simulink model "SailingYachtModel"  (R2022b)
settings: Solver=ode3  StartTime=0.0  StopTime=250  FixedStep=0.05  RelTol=1e-3  EnableMultiTasking=on
undefined symbols (not defined in the file or in its folder): par, Waypoints
libraries: simulink x1, vrlib x1
settings Model: Creator=Administrator  LastModifiedBy=ruben
settings SolverCC: AlgebraicLoopSolver=TrustRegion  AutoInsertRateTranBlk=on
settings DataIOCC: LimitDataPoints=on  SaveFormat=Array  SignalLoggingSaveFormat=ModelDataLogs  ReturnWorkspaceOutputs=off
settings OptimizationCC: ExpressionDepthLimit=2147483647  InitFltsAndDblsToZero=on  LifeSpan=inf
settings DebuggingCC: SaveWithParameterizedLinksMsg=none  UnderspecifiedInitializationDetection=Classic  MergeDetectMultiDrivingBlocksExec=none  SignalResolutionControl=TryResolveAllWithWarning  SolverPrmCheckMsg=warning  MultiTaskDSMMsg=warning  MultiTaskCondExecSysMsg=none  FcnCallInpInsideContextMsg=warning  UnconnectedInputMsg=warning  UnconnectedOutputMsg=warning  UnconnectedLineMsg=warning  StateNameClashWarn=warning  SFUnexpectedBacktrackingDiag=warning  SFNoUnconditionalDefaultTransitionDiag=warning  SFExecutionAtInitializationDiag=none  SFMachineParentedDataDiag=warning  ArithmeticOperatorsInVariantConditions=warning
settings HardwareCC: ProdBitPerPointer=32  ProdBitPerSizeT=32  ProdBitPerPtrDiffT=32  ProdLargestAtomicFloat=None  ProdIntDivRoundTo=Undefined  ProdEndianess=Unspecified  ProdWordSize=32  ProdHWDeviceType=32-bit Generic
settings ModelReferenceCC: PropagateSignalLabelsOutOfModel=off
settings SFSimCC: SimUseLocalCustomCode=off  CustomCodeUndefinedFunction=UseInterfaceOnly
settings RTWCC: RTWUseLocalCustomCode=off
settings CodeAppCC: StateflowObjectComments=on
settings GRTTargetCC: TargetFcnLib=ansi_tfl_tmw.mat  TargetLangStandard=C89/C90 (ANSI)  CombineOutputUpdateFcns=off  GRTInterface=on
settings ConfigComp: CovMetricSettings=dw  CovSaveCumulativeToWorkspaceVar=on  CovSaveSingleToWorkspaceVar=on  CovExternalEMLEnable=off

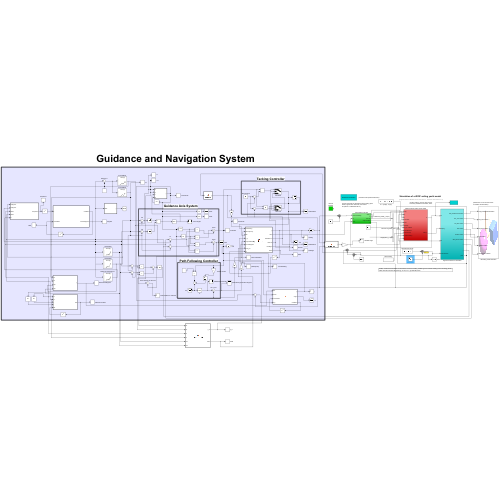
[thumbnail: Simulink's stored preview of the top-level diagram]
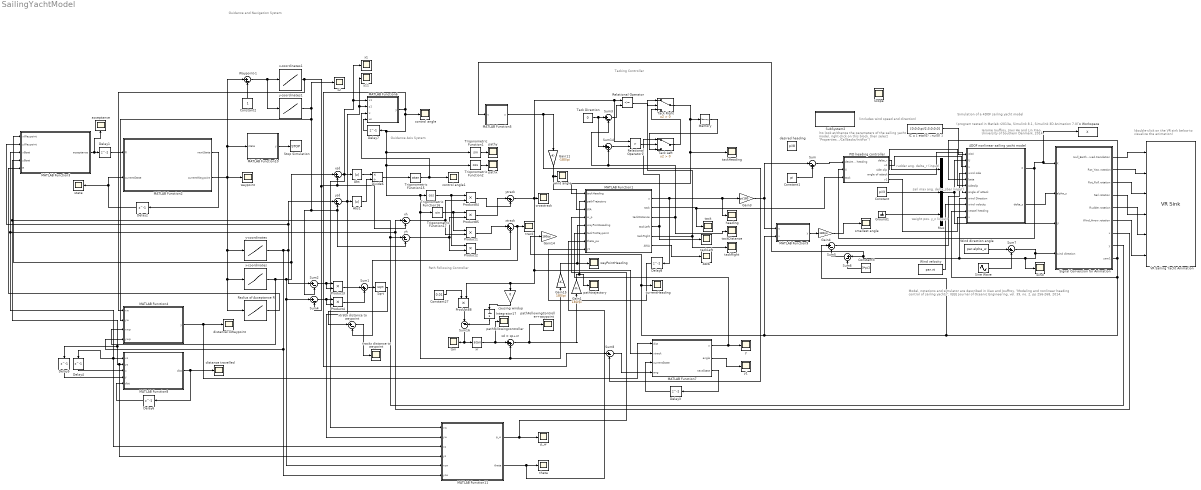
== system SailingYachtModel ==
  note: Guidance Axis System
  note: (includes wind speed and direction)
  note: (program tested in Matlab r2013a, Simulink 8.1, Simulink 3D Animation 7.0)
  note: (double-click on the VR sink below
      | to visualize the animation)
  note: Jerome Jouffroy, Jiaxi He and Lin Xiao,
      | University of Southern Denmark, 2014.
  note: Model, notations and simulator are described in Xiao and Jouffroy, "Modeling and nonlinear heading control of sailing yachts",
      | IEEE Journal of Oceanic Engineering, vol. 39, no. 2, pp 256-268, 2014.
  note: (to look at/change the parameters of the sailing yacht
      | model, right-click on this block, then select
      | "Properties.../Callbacks/InitFcn")
  note: weight pos. y_c (input)
  note: rudder ang. delta_r (input)
  note: sail max ang. delta_sbar (input)
  note: Simulation of a 4DOF sailing yacht model
  note: Path Following Controller
  note: Tacking Controller
  note: Guidance and Navigation System
  4DOF nonlinear sailing yacht model : Subsystem
  AWA : Scope
  Abs : Abs  SaturateOnIntegerOverflow=off
  Abs1 : Abs  SaturateOnIntegerOverflow=off
  Constant : Constant  Value=pi/3
  Constant1 : Constant  Value=pi
  Constant2 : Constant
  Constant27 : Constant  Value=0.01
  Constant3 : Constant  Value=3*pi/2
  Delay{1..8} (8 alike) : Delay  DelayLength=1
  Divide6 : Product  Inputs=*/
  Gain{1,4,14..15} (4 alike) : Gain  Gain=180/pi
  Gain11 : Gain  Gain=-180/pi
  Gain3 : Gain  Gain=pi/180
  Ground1 : Ground
  IC = [ eta(0) ; nu(0) ] : Constant  Value=[0;0;0;pi/2;3;0;0;0]
  Integrator17 : Integrator  LimitOutput=on  UpperSaturationLimit=10  LowerSaturationLimit=-10
  MATLAB Function1 : MATLAB Function  TreatAsAtomicUnit=on
  MATLAB Function10 : MATLAB Function  TreatAsAtomicUnit=on
  MATLAB Function11 : MATLAB Function  TreatAsAtomicUnit=on
  MATLAB Function2 : MATLAB Function  TreatAsAtomicUnit=on
  MATLAB Function3 : MATLAB Function  TreatAsAtomicUnit=on
  MATLAB Function4 : MATLAB Function  TreatAsAtomicUnit=on
  MATLAB Function5 : MATLAB Function  TreatAsAtomicUnit=on
  MATLAB Function6 : MATLAB Function  TreatAsAtomicUnit=on
  MATLAB Function7 : MATLAB Function  TreatAsAtomicUnit=on
  MATLAB Function8 : MATLAB Function  TreatAsAtomicUnit=on
  MATLAB Function9 : MATLAB Function  TreatAsAtomicUnit=on
  Memory : Memory
  Mux : Mux  Inputs=3
  PID heading controller : Subsystem
  Product{1..4,84..85,88} (7 alike) : Product
  Radius of Acceptance R : Lookup_n-D  NumberOfTableDimensions=1  BreakpointsForDimension1=Waypoints.number  Table=Waypoints.R  InterpMethod=Cubic spline  ExtrapMethod=Cubic spline  InternalRulePriority=Speed  RndMeth=Simplest
  Relational Operator : RelationalOperator  Operator=<=  OutDataTypeStr=boolean  RndMeth=Simplest  InputSameDT=off
  Relational Operator1 : RelationalOperator  Operator=>  OutDataTypeStr=boolean  RndMeth=Simplest  InputSameDT=off
  Signal Conversion for Animation : Subsystem
  Sine Wave : Sin  Amplitude=pi/14  Frequency=0.1  SampleTime=0
  Sqrt : Sqrt
  Stop Simulation : Stop
  SubSystem2 : Subsystem  InitFcn=|
      | global par
      | par.m = 25900;                         % (kg),mass of the vehicle
      | par.Ixx = 133690;          
      | par.Izz = 24760;      
      | par.Ixz = 2180;                        % moment of inertia
      | par.a11 = 970;   
      | par.a22 = 17430; 
      | par.a44 = 106500;
      | par.a66 = 101650;
      | par.a24 = -13160;
      | par.a26 = -6190; 
      | par.a46 = 4730;                        % (kg),added mass coef.
      | 
      | par.vt = 15;                           % the norm of wind velocity
      | par.alpha_w = -(-pi/2+pi/18);                      % the direction of wind (coming from the north, ie going south)
      | 
      | par.rho_a = 1.2;                       % (kg/m^3), air density
      | par.As = 170;                          % (m^2), sail area
      | par.h0 = 0.0005;                       % (m), roughness height
      | par.h1 = 11.58;                        % (m), reference height
      | par.z_s = -11.58;                      % (m), (x,y,z) is the CoE
      | par.xs = 0;
      | par.ys = 0;
      | par.zs = -11.58;                       % (m), (x,y,z) is the CoE
      | par.Xce = 0.6;                         % (m), distance along the mast to the CoE
      | par.Xm = 0.3;                          % (m), x-coordinate of the mast 
      | 
      | par.rho_w = 1025;                      % (kg/m^3), water density
      | par.Ar = 1.17;                         % (m^2), rudder area
      | par.d_r = 1.9;                         % rudder draft
      | par.zeta_r = 0.8;                      % rudder efficiency
      | par.x_r = -8.2;
      | par.z_r = -0.78;                       % (m), (x,y,z) is the CoE
      | par.xr = -8.2;
      | par.yr = 0;
      | par.zr = -0.78;                        % (m), (x,y,z) is the CoE
      | 
      | par.Ak = 8.7;                          % (m^2), keel area
      | par.d_k = 2.49;                        % keel draft
      | par.zeta_k = 0.7;                      % keel efficiency
      | par.x_k = 0;
      | par.z_k = -0.58;                       % (m), (x,y,z) is the CoE
      | par.xk = 0;
      | par.yk = 0;
      | par.zk = -0.58;                        % (m), (x,y,z) is the CoE
      | 
      | par.x_h = 0;
      | par.z_h = -1.18;                       % (m), (x,y,z) is the CoE
      | par.xh = 0;
      | par.yh = 0;
      | par.zh = -1.18;                        % (m), (x,y,z) is the CoE
      | 
      | par.w_c = 60000;                       % (N), crew weight 20000
      | par.x_c = -8;                          % (m), crew position
      | par.y_bm = 3.6;                        % (m), yacht beam
      | 
      | par.a = -5.89;
      | par.b = 8160;
      | par.c = 120000;
      | par.d = 50000;
      mask Display: disp('Parameter Initialization')
  Sum : Sum  Inputs=|-+  SaturateOnIntegerOverflow=on
  Sum1 : Sum  Inputs=|++
  Sum14 : Sum  Inputs=|++
  Sum16 : Sum  Inputs=|--
  Sum{2..4,8} (4 alike) : Sum  Inputs=|+-
  Sum5 : Sum  Inputs=|+-  SaturateOnIntegerOverflow=on
  Sum6 : Sum  Inputs=|+-  SaturateOnIntegerOverflow=on
  Sum7 : Sum  Inputs=|+-  SaturateOnIntegerOverflow=on
  Tack Direction : Constant  Value=0
  Tack Left : Switch  Criteria=u2 > Threshold  SaturateOnIntegerOverflow=off  InputSameDT=off
  Tack Right : Switch  Criteria=u2 > Threshold  SaturateOnIntegerOverflow=off  InputSameDT=off
  To Workspace : ToWorkspace  VariableName=X  SaveFormat=Structure With Time  SampleTime=-1
  Trigonometric Function1 : Trigonometry
  Trigonometric Function15 : Trigonometry  Operator=atan
  Trigonometric Function16 : Trigonometry  Operator=cos
  Trigonometric Function17 : Trigonometry
  Trigonometric Function2 : Trigonometry  Operator=cos
  VR Sailing Yacht Animation : vrlib/VR Sink  InstantiateOnLoad=on  SampleTime=-1  ViewEnable=on  RemoteChange=off  RemoteView=off  FieldsWritten=Hull_EarthFixed.translation.3.1.1.double#Rot_Yaw.rotation.4.1.1.double#Rot_Roll.rotation.4.1.1.double#Sail.rotation.4.1.1.double#Rudder.rotation.4.1.1.double#Wind_Arrow.rotation.4.1.1.double  WorldFileName=SailingYachtAnimation.wrl  WorldDescription=Sailing Yacht VR animation  AutoView=on  VideoDimensions=[]  AllowVariableSize=off  FigureProperties="{'Position', 'Name', 'Viewpoint', 'CameraBound', 'CameraDirection', 'CameraPosition', 'CameraUpVector', 'ZoomFactor', 'Antialiasing', 'Headlight', 'Lighting', 'NavPanel', 'Sound', 'StatusBar', 'Stereo3D', 'Stereo3DCameraOffset', 'Stereo3DHIT', 'ToolBar', 'Textures', 'Transparency', 'Triad', 'Wireframe', 'NavZones', 'NavMode', 'NavSpeed', 'CaptureFileFormat', 'CaptureFileName', 'Record2DCompressMethod', 'Record2DCompressQuality', 'Record2D', 'Record2DFileName', 'Record2DFPS'; [2.0000000000000000e+00   8.4000000000000000e+01   9.5800000000000000e+02   8.9600000000000000e+02], 'Sailing Yacht VR animation', 'Stern', 'on', [2.8705425156036607e-01   0.0000000000000000e+00  -9.5791432636803509e-01], [-1.9182625747857539e+01   1.3000000000000000e+01   3.6417716435568920e+01], [0.0000000000000000e+00   1.0000000000000000e+00   0.0000000000000000e+00], [1.0000000000000000e+00], 'on', 'on', 'on', 'halfbar', 'on', 'on', 'off', [1.0000000149011612e-01], [0.0000000000000000e+00], 'on', 'on', 'on', 'none', 'off', 'off', 'walk', 'normal', 'tif', '%f_anim_%n.tif', 'auto', [7.5000000000000000e+01], 'on', '%f_anim_%n.avi', [1.5000000000000000e+01]}"
  Waypoint-1 : Sum  Inputs=|+-
  Wind direction angle : Constant  Value=par.alpha_w
  Wind velocity : Constant  Value=par.vt
  acceptance : Scope
  causing windup : Gain  Gain=0
  control angle : Scope
  control angle1 : Scope
  crosstrack : Scope
  currentHeading : Scope
  desired heading : Constant  Value=pi/8
  distance travelled : Scope
  distanceToWaypoint : Scope
  heading : Scope
  p_w : Scope
  "pathFollowingController+waypoint " : Scope
  pathfollowingcontroller : Scope
  pathtrajectory : Scope
  pathx : Scope
  pathy : Scope
  smallest angle : Scope
  state : Scope
  tack : Scope
  tackDistance : Scope
  tackHeading : Scope
  tackLeft : Scope
  tackRight : Scope
  tan : Scope
  theta : Scope
  track : Scope
  trackx distance to waypoint : Scope
  wayPointHeading : Scope
  waypoint : Scope
  wind : Scope
  wind angle : Scope
  x-coordinates : Lookup_n-D  NumberOfTableDimensions=1  BreakpointsForDimension1=Waypoints.number  Table=Waypoints.x  InterpMethod=Cubic spline  ExtrapMethod=Cubic spline  InternalRulePriority=Speed  RndMeth=Simplest
  x-coordinates1 : Lookup_n-D  NumberOfTableDimensions=1  BreakpointsForDimension1=Waypoints.number  Table=Waypoints.x  InterpMethod=Cubic spline  ExtrapMethod=Cubic spline  InternalRulePriority=Speed  RndMeth=Simplest
  x1 : Scope
  x2 : Scope
  xd = xp+xr : Sum  Inputs=|++
  xh : Sum  Inputs=|+-
  xr : Trigonometry  Operator=atan
  xsd : Sum  Inputs=|+-
  xtrack : Sum  Inputs=|++
  xtrack distance to waypoint : Sum  Inputs=|+-
  y : Scope
  y-coordinates : Lookup_n-D  NumberOfTableDimensions=1  BreakpointsForDimension1=Waypoints.number  Table=Waypoints.y  InterpMethod=Cubic spline  ExtrapMethod=Cubic spline  InternalRulePriority=Speed  RndMeth=Simplest
  y-coordinates1 : Lookup_n-D  NumberOfTableDimensions=1  BreakpointsForDimension1=Waypoints.number  Table=Waypoints.y  InterpMethod=Cubic spline  ExtrapMethod=Cubic spline  InternalRulePriority=Speed  RndMeth=Simplest
  y1 : Scope
  y11 : Scope
  yh : Sum  Inputs=|+-
  ysd : Sum  Inputs=|+-
  ytrack : Sum  Inputs=|-+
  Scope : Scope
  wires:
  Constant/1 -> Mux/2
  IC = [ eta(0) ; nu(0) ]/1 -> 4DOF nonlinear sailing yacht model/1(X(0))
  Mux/1 -> Signal Conversion for Animation/3(U), 4DOF nonlinear sailing yacht model/2(U)
  4DOF nonlinear sailing yacht model/1(X) -> Signal Conversion for Animation/1(X), To Workspace/1, PID heading controller/2(X)
  PID heading controller/1(delta_r) -> Mux/1
  Ground1/1 -> Mux/3
  4DOF nonlinear sailing yacht model/2(delta_s) -> Signal Conversion for Animation/2(alpha_s)
  Signal Conversion for Animation/1(Hull_EarthFixed.translation) -> VR Sailing Yacht Animation/1
  Signal Conversion for Animation/2(Rot_Yaw.rotation) -> VR Sailing Yacht Animation/2
  Signal Conversion for Animation/4(Sail.rotation) -> VR Sailing Yacht Animation/4
  Signal Conversion for Animation/3(Rot_Roll.rotation) -> VR Sailing Yacht Animation/3
  Signal Conversion for Animation/5(Rudder.rotation) -> VR Sailing Yacht Animation/5
  Signal Conversion for Animation/6(Wind_Arrow.rotation) -> VR Sailing Yacht Animation/6
  Delay1/1 -> MATLAB Function2/1(R)
  Delay2/1 -> MATLAB Function2/2(currentState), state/1
  Trigonometric Function15/1 -> control angle1/1, MATLAB Function6/3(u)
  ysd/1 -> MATLAB Function11/2(yw), y11/1, MATLAB Function6/2(y1), Abs1/1
  Trigonometric Function17/1 -> Product1/1, Product85/1
  Product85/1 -> ytrack/1
  Product84/1 -> ytrack/2
  Trigonometric Function16/1 -> Product2/1, Product84/1
  xh/1 -> Product84/2, Product1/2
  xsd/1 -> MATLAB Function11/1(xw), MATLAB Function6/1(x1), x1/1, Abs/1
  yh/1 -> Product85/2, Product2/2
  Divide6/1 -> Trigonometric Function15/1
  MATLAB Function2/2(currentWaypoint) -> MATLAB Function10/1(state), Waypoint-1/1, waypoint/1, Radius of Acceptance R/1, x-coordinates/1, y-coordinates/1
  Waypoint-1/1 -> x-coordinates1/1, y-coordinates1/1
  Constant2/1 -> Waypoint-1/2
  MATLAB Function2/1(nextState) -> Delay2/1
  y-coordinates/1 -> MATLAB Function11/6(ycw), MATLAB Function4/4(ywp), MATLAB Function3/2(yWaypoint), ysd/1, Sum2/1
  x-coordinates/1 -> MATLAB Function4/3(xwp), MATLAB Function11/5(xcw), Sum4/1, xsd/1, MATLAB Function3/1(xWaypoint)
  y-coordinates1/1 -> MATLAB Function4/2(yw), yh/2, ysd/2, Sum2/2, x2/1
  x-coordinates1/1 -> MATLAB Function4/1(xw), Sum4/2, xh/2, xsd/2
  MATLAB Function6/1(y) -> Trigonometric Function1/1, Trigonometric Function2/1, Trigonometric Function17/1, xd = xp+xr/2, Gain15/1, Trigonometric Function16/1, Delay7/1, control angle/1, Sum8/1
  Product88/1 -> Sum16/1
  Sum16/1 -> xr/1, tan/1
  Constant27/1 -> Product88/1
  xr/1 -> xd = xp+xr/1, pathfollowingcontroller/1
  Gain15/1 -> MATLAB Function1/5(wayPointHeading), wayPointHeading/1
  Signal Conversion for Animation/7(x) -> xh/1, MATLAB Function11/3(xs), MATLAB Function8/1(xs), Delay4/1, MATLAB Function3/3(xBoat)
  Signal Conversion for Animation/8(y) -> yh/1, MATLAB Function3/4(yBoat), MATLAB Function11/4(ys), MATLAB Function8/2(ys), Delay5/1
  Sum3/1 -> Relational Operator/2
  Tack Right/1 -> Memory/1, tackHeading/1, MATLAB Function1/1(tackHeading)
  Memory/1 -> Tack Left/3
  Tack Left/1 -> Tack Right/3
  Relational Operator1/1 -> Tack Left/2
  Tack Direction/1 -> Sum14/1, Sum3/1
  Relational Operator/1 -> Tack Right/2
  Sum14/1 -> Relational Operator1/2
  MATLAB Function1/3(tackDistance) -> Sum3/2, Sum14/2, tackDistance/1
  MATLAB Function5/1(y) -> Sum8/2, Gain11/1
  Gain11/1 -> MATLAB Function1/3(WA), wind angle/1
  MATLAB Function1/4(tackLeft) -> Tack Left/1, tackLeft/1
  MATLAB Function1/5(tackRight) -> Tack Right/1, tackRight/1
  MATLAB Function1/1(y) -> Delay8/1, heading/1, Gain3/1
  Radius of Acceptance R/1 -> MATLAB Function3/5(R)
  MATLAB Function3/1(acceptance) -> acceptance/1, Delay1/1
  causing windup/1 -> Integrator17/1
  Integrator17/1 -> Sum16/2
  xd = xp+xr/1 -> "pathFollowingController+waypoint "/1, Gain1/1
  ytrack/1 -> Product88/2, causing windup/1, MATLAB Function7/2(xtrack), crosstrack/1, Relational Operator1/1, Relational Operator/1
  MATLAB Function1/2(tack) -> tack/1, PID heading controller/3(tack)
  Gain1/1 -> MATLAB Function1/2(pathTrajectory), pathtrajectory/1
  MATLAB Function4/1(y) -> MATLAB Function7/1(dist), distanceToWaypoint/1
  MATLAB Function7/1(y) -> y/1, MATLAB Function1/6(tackToWaypoint)
  MATLAB Function7/2(angle) -> y1/1
  MATLAB Function7/3(nextState) -> Delay3/1
  Delay3/1 -> MATLAB Function7/3(currentState)
  Product1/1 -> xtrack/1
  Product2/1 -> xtrack/2
  xtrack/1 -> xtrack distance to waypoint/2, track/1
  Product3/1 -> Sum1/1
  Product4/1 -> Sum1/2
  Sum1/1 -> Sqrt/1
  Sum4/1 -> Product4/2, Product4/1
  Sum2/1 -> Product3/1, Product3/2
  Sqrt/1 -> xtrack distance to waypoint/1
  xtrack distance to waypoint/1 -> trackx distance to waypoint/1
  Delay4/1 -> MATLAB Function8/3(x)
  Delay5/1 -> MATLAB Function8/4(y)
  MATLAB Function8/1(dist) -> distance travelled/1, Delay6/1
  Delay6/1 -> MATLAB Function8/5("dist ")
  PID heading controller/2(u1) -> 4DOF nonlinear sailing yacht model/3(u)
  Gain3/1 -> MATLAB Function9/1(u), Sum/1
  Sum5/1 -> 4DOF nonlinear sailing yacht model/4(wind side)
  Constant3/1 -> Sum6/2
  Sum6/1 -> Sum5/2
  Signal Conversion for Animation/9(yaw1) -> 4DOF nonlinear sailing yacht model/10(vessel heading), Sum5/1, MATLAB Function9/2(v), Gain14/1, currentHeading/1, 4DOF nonlinear sailing yacht model/5(beta)
  MATLAB Function9/1(y) -> Gain4/1
  Gain4/1 -> smallest angle/1
  Trigonometric Function1/1 -> pathy/1
  Trigonometric Function2/1 -> pathx/1
  Constant1/1 -> Sum/2
  Sum/1 -> PID heading controller/1(desired heading)
  Abs1/1 -> Divide6/2
  Abs/1 -> Divide6/1
  Delay7/1 -> MATLAB Function6/4(us)
  MATLAB Function10/1(y) -> Stop Simulation/1
  Wind direction angle/1 -> Sum7/1
  Sum7/1 -> wind/1, MATLAB Function5/1(u), Sum6/1, 4DOF nonlinear sailing yacht model/8(wind Direction), Signal Conversion for Animation/4(wind direction)
  Sum8/1 -> MATLAB Function7/4(ang)
  PID heading controller/3(side slip) -> 4DOF nonlinear sailing yacht model/6(sideslip)
  PID heading controller/4(angle of attack) -> 4DOF nonlinear sailing yacht model/7(angle of attack)
  PID heading controller/5(v1) -> 4DOF nonlinear sailing yacht model/11(v)
  Wind velocity/1 -> 4DOF nonlinear sailing yacht model/9(wind velocity)
  Sine Wave/1 -> Sum7/2
  MATLAB Function1/6(AWA) -> AWA/1
  MATLAB Function11/1(p_w) -> MATLAB Function1/4(w_p), p_w/1
  MATLAB Function11/2(theta) -> MATLAB Function1/7(theta_pw), theta/1
  Delay8/1 -> MATLAB Function1/8(ys)

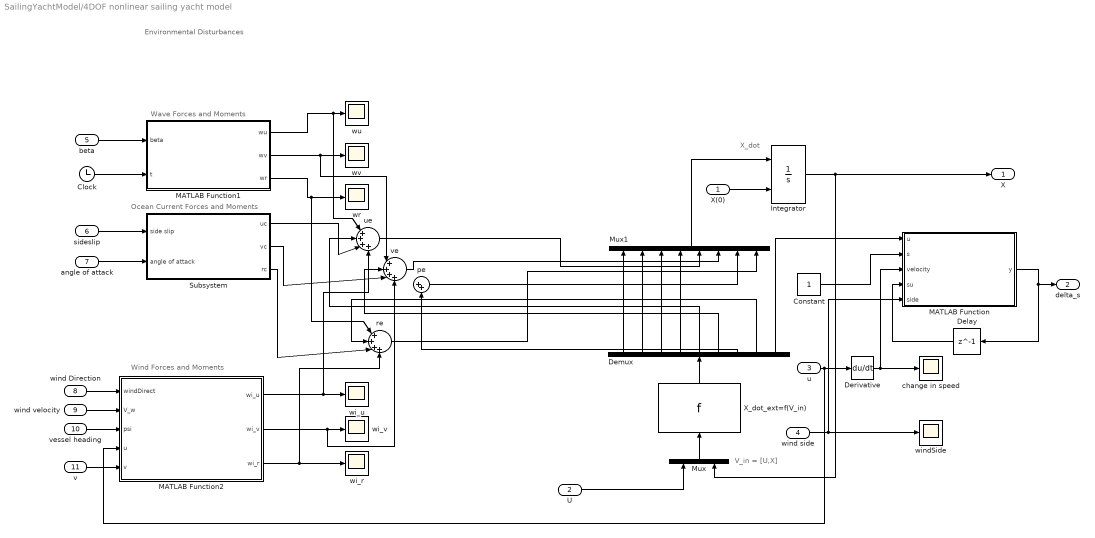
== system SailingYachtModel/4DOF nonlinear sailing yacht model ==
  note: Wave Forces and Moments
  note: Environmental Disturbances
  note: X_dot
  note: V_in = [U,X]
  note: Ocean Current Forces and Moments
  note: Wind Forces and Moments
  X(0) : Inport
  U : Inport  Port=2
  u : Inport  Port=3
  wind side : Inport  Port=4
  beta : Inport  Port=5
  sideslip : Inport  Port=6
  angle of attack : Inport  Port=7
  wind Direction : Inport  Port=8
  wind velocity : Inport  Port=9
  vessel heading : Inport  Port=10
  v : Inport  Port=11
  Clock : Clock
  Constant : Constant
  Delay : Delay  DelayLength=1  InitialCondition=0
  Demux : Demux  Outputs=9
  Derivative : Derivative
  Integrator : Integrator  InitialConditionSource=external  InitialCondition=[0;0;0;pi;1;0;0;0]
  MATLAB Function : MATLAB Function  TreatAsAtomicUnit=on
  MATLAB Function1 : MATLAB Function  TreatAsAtomicUnit=on
  MATLAB Function2 : MATLAB Function  TreatAsAtomicUnit=on
  Mux : Mux  Inputs=2
  Mux1 : Mux  Inputs=8
  Subsystem : Subsystem
  X_dot_ext=f(V_in) : MATLABFcn  MATLABFcn=f  OutputDimensions=9
  change in speed : Scope
  pe : Sum  Inputs=|++
  re : Sum  Inputs=|++++
  ue : Sum  Inputs=|++++
  ve : Sum  Inputs=|++++
  wi_r : Scope
  wi_u : Scope
  wi_v : Scope
  windSide : Scope
  wr : Scope
  wu : Scope
  wv : Scope
  X : Outport
  delta_s : Outport  Port=2
  wires:
  X(0)/1 -> Integrator/2
  Mux/1 -> X_dot_ext=f(V_in)/1
  U/1 -> Mux/1
  Integrator/1 -> X/1, Mux/2
  X_dot_ext=f(V_in)/1 -> Demux/1
  Demux/4 -> Mux1/4
  Demux/3 -> Mux1/3
  Demux/2 -> Mux1/2
  Demux/1 -> Mux1/1
  Mux1/1 -> Integrator/1
  Demux/9 -> MATLAB Function/1(u)
  MATLAB Function/1(y) -> Delay/1, delta_s/1
  Constant/1 -> MATLAB Function/2(s)
  u/1 -> MATLAB Function2/4(u), Derivative/1
  Derivative/1 -> change in speed/1, MATLAB Function/3(velocity)
  Delay/1 -> MATLAB Function/4(su)
  wind side/1 -> MATLAB Function/5(side), windSide/1
  Demux/5 -> ue/2
  Demux/6 -> ve/2
  Demux/7 -> pe/2
  Demux/8 -> re/2
  ue/1 -> Mux1/5
  ve/1 -> Mux1/6
  pe/1 -> Mux1/7
  re/1 -> Mux1/8
  Clock/1 -> MATLAB Function1/2(t)
  MATLAB Function1/1(wu) -> ue/1, wu/1
  MATLAB Function1/2(wv) -> ve/1, wv/1
  MATLAB Function1/3(wr) -> re/1, wr/1
  beta/1 -> MATLAB Function1/1(beta)
  Subsystem/3(rc) -> re/3
  sideslip/1 -> Subsystem/1(side slip)
  angle of attack/1 -> Subsystem/2(angle of attack)
  Subsystem/1(uc) -> ue/3
  Subsystem/2(vc) -> ve/3
  MATLAB Function2/1(wi_u) -> ue/4, wi_u/1
  MATLAB Function2/3(wi_r) -> wi_r/1, re/4
  wind Direction/1 -> MATLAB Function2/1(windDirect)
  wind velocity/1 -> MATLAB Function2/2(V_w)
  vessel heading/1 -> MATLAB Function2/3(psi)
  v/1 -> MATLAB Function2/5(v)
  MATLAB Function2/2(wi_v) -> ve/4, wi_v/1

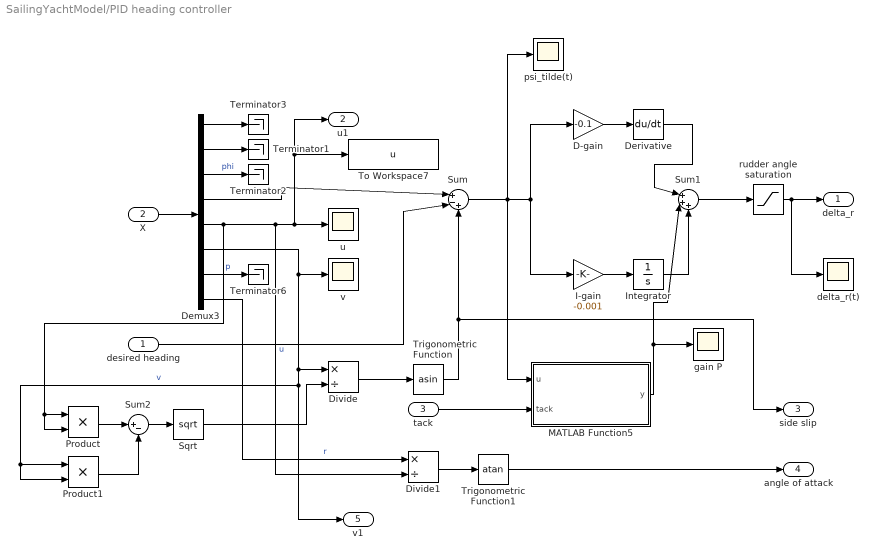
== system SailingYachtModel/PID heading controller ==
  desired heading : Inport
  X : Inport  Port=2
  tack : Inport  Port=3
  D-gain : Gain  Gain=-0.1
  Demux3 : Demux  Outputs=8
  Derivative : Derivative
  Divide : Product  Inputs=*/
  Divide1 : Product  Inputs=*/
  I-gain : Gain  Gain=-0.001
  Integrator : Integrator
  MATLAB Function5 : MATLAB Function  TreatAsAtomicUnit=on
  Product : Product
  Product1 : Product
  Sqrt : Sqrt  IntermediateResultsDataTypeStr=double
  Sum : Sum  Inputs=|+-+  SaturateOnIntegerOverflow=on
  Sum1 : Sum  Inputs=|+++  SaturateOnIntegerOverflow=on
  Sum2 : Sum  Inputs=|+-  SaturateOnIntegerOverflow=on
  Terminator{1..3,6} (4 alike) : Terminator
  To Workspace7 : ToWorkspace  VariableName=u  SaveFormat=Timeseries  SampleTime=-1
  Trigonometric Function : Trigonometry  Operator=asin
  Trigonometric Function1 : Trigonometry  Operator=atan
  delta_r(t) : Scope
  gain P : Scope
  psi_tilde(t) : Scope
  rudder angle saturation : Saturate  UpperLimit=pi/6  LowerLimit=-pi/6  LinearizeAsGain=off
  u : Scope
  v : Scope
  delta_r : Outport
  u1 : Outport  Port=2
  side slip : Outport  Port=3
  angle of attack : Outport  Port=4
  v1 : Outport  Port=5
  wires:
  X/1 -> Demux3/1
  Demux3/1 -> Terminator3/1
  Demux3/2 -> Terminator1/1
  Demux3/3 -> Terminator2/1  "phi"
  Demux3/5 -> u1/1, To Workspace7/1, u/1, Divide1/2, Product/2, Product/1  "u"
  Demux3/6 -> v1/1, Product1/2, Product1/1, Divide/1, v/1  "v"
  Demux3/7 -> Terminator6/1  "p"
  Demux3/8 -> Divide1/1  "r"
  Sum/1 -> MATLAB Function5/1(u), I-gain/1, D-gain/1, psi_tilde(t)/1
  desired heading/1 -> Sum/2
  rudder angle saturation/1 -> delta_r(t)/1, delta_r/1
  Sum1/1 -> rudder angle saturation/1
  I-gain/1 -> Integrator/1
  D-gain/1 -> Derivative/1
  Derivative/1 -> Sum1/1
  MATLAB Function5/1(y) -> gain P/1, Sum1/2
  Integrator/1 -> Sum1/3
  Demux3/4 -> Sum/1
  tack/1 -> MATLAB Function5/2(tack)
  Divide/1 -> Trigonometric Function/1
  Trigonometric Function/1 -> side slip/1, Sum/3
  Trigonometric Function1/1 -> angle of attack/1
  Divide1/1 -> Trigonometric Function1/1
  Sum2/1 -> Sqrt/1
  Product/1 -> Sum2/1
  Product1/1 -> Sum2/2
  Sqrt/1 -> Divide/2

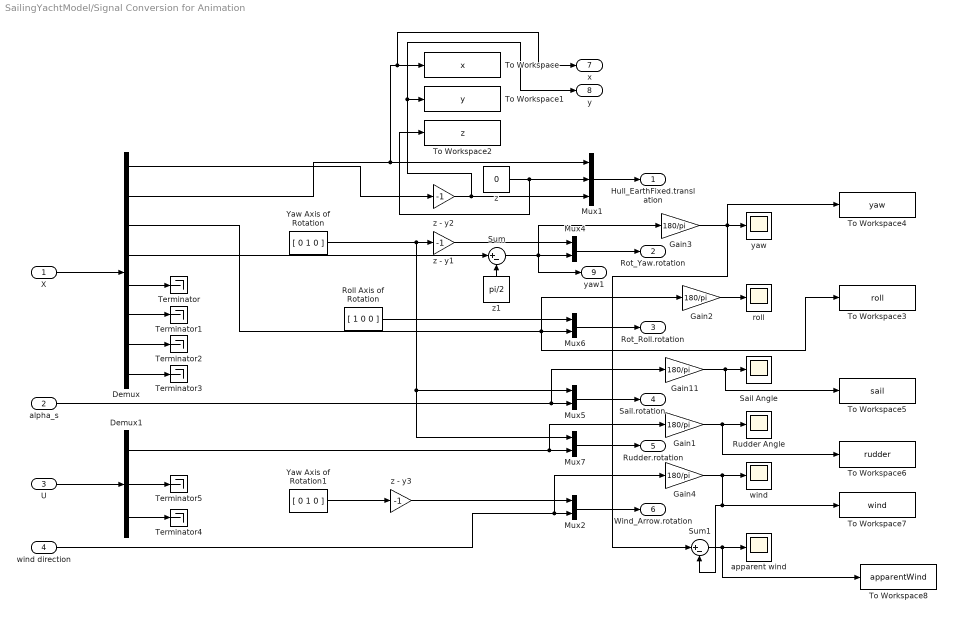
== system SailingYachtModel/Signal Conversion for Animation ==
  X : Inport
  alpha_s : Inport  Port=2
  U : Inport  Port=3
  wind direction : Inport  Port=4
  Demux : Demux  Outputs=8
  Demux1 : Demux  Outputs=3
  Gain{1..4,11} (5 alike) : Gain  Gain=180/pi
  Mux1 : Mux  Inputs=3
  Mux{2,4..7} (5 alike) : Mux  Inputs=2
  Roll Axis of Rotation : Constant  Value=[ 1 0 0 ]
  Rudder Angle : Scope
  Sail Angle : Scope
  Sum : Sum  Inputs=|+-  SaturateOnIntegerOverflow=on
  Sum1 : Sum  Inputs=|+-  SaturateOnIntegerOverflow=on
  Terminator{,1..5} (6 alike) : Terminator
  To Workspace : ToWorkspace  VariableName=x  SaveFormat=Timeseries  SampleTime=-1
  To Workspace1 : ToWorkspace  VariableName=y  SaveFormat=Timeseries  SampleTime=-1
  To Workspace2 : ToWorkspace  VariableName=z  SaveFormat=Timeseries  SampleTime=-1
  To Workspace3 : ToWorkspace  VariableName=roll  SaveFormat=Timeseries  SampleTime=-1
  To Workspace4 : ToWorkspace  VariableName=yaw  SaveFormat=Timeseries  SampleTime=-1
  To Workspace5 : ToWorkspace  VariableName=sail  SaveFormat=Timeseries  SampleTime=-1
  To Workspace6 : ToWorkspace  VariableName=rudder  SaveFormat=Timeseries  SampleTime=-1
  To Workspace7 : ToWorkspace  VariableName=wind  SaveFormat=Timeseries  SampleTime=-1
  To Workspace8 : ToWorkspace  VariableName=apparentWind  SaveFormat=Timeseries  SampleTime=-1
  Yaw Axis of Rotation : Constant  Value=[ 0 1 0 ]
  Yaw Axis of Rotation1 : Constant  Value=[ 0 1 0 ]
  apparent wind : Scope
  roll : Scope
  wind : Scope
  yaw : Scope
  z : Constant  Value=0
  z - y1 : Gain  Gain=-1
  z - y2 : Gain  Gain=-1
  z - y3 : Gain  Gain=-1
  z1 : Constant  Value=pi/2
  Hull_EarthFixed.translation : Outport
  Rot_Yaw.rotation : Outport  Port=2
  Rot_Roll.rotation : Outport  Port=3
  Sail.rotation : Outport  Port=4
  Rudder.rotation : Outport  Port=5
  Wind_Arrow.rotation : Outport  Port=6
  x : Outport  Port=7
  y : Outport  Port=8
  yaw1 : Outport  Port=9
  wires:
  Yaw Axis of Rotation/1 -> Mux5/1, Mux7/1, z - y1/1
  Sum/1 -> Gain3/1, yaw1/1, Mux4/2
  Roll Axis of Rotation/1 -> Mux6/1
  Demux/3 -> Gain2/1, To Workspace3/1, Mux6/2
  alpha_s/1 -> Gain11/1, Mux5/2
  Demux/1 -> z - y2/1
  z - y2/1 -> y/1, To Workspace1/1, Mux1/3
  Demux/2 -> Mux1/1, x/1, To Workspace/1
  z - y1/1 -> Mux4/1
  Mux1/1 -> Hull_EarthFixed.translation/1
  Demux/5 -> Terminator/1
  Demux/6 -> Terminator1/1
  Demux/7 -> Terminator2/1
  Demux/8 -> Terminator3/1
  X/1 -> Demux/1
  Demux1/3 -> Terminator4/1
  Demux1/2 -> Terminator5/1
  U/1 -> Demux1/1
  Demux1/1 -> Gain1/1, Mux7/2
  Mux7/1 -> Rudder.rotation/1
  Mux5/1 -> Sail.rotation/1
  Mux4/1 -> Rot_Yaw.rotation/1
  Yaw Axis of Rotation1/1 -> z - y3/1
  z - y3/1 -> Mux2/1
  wind direction/1 -> Gain4/1, Mux2/2
  Mux2/1 -> Wind_Arrow.rotation/1
  Mux6/1 -> Rot_Roll.rotation/1
  z/1 -> Mux1/2, To Workspace2/1
  Demux/4 -> Sum/1
  z1/1 -> Sum/2
  Gain11/1 -> To Workspace5/1, Sail Angle/1
  Gain1/1 -> To Workspace6/1, Rudder Angle/1
  Gain2/1 -> roll/1
  Gain3/1 -> Sum1/1, To Workspace4/1, yaw/1
  Gain4/1 -> Sum1/2, To Workspace7/1, wind/1
  Sum1/1 -> To Workspace8/1, apparent wind/1

== system SailingYachtModel/SubSystem2 ==

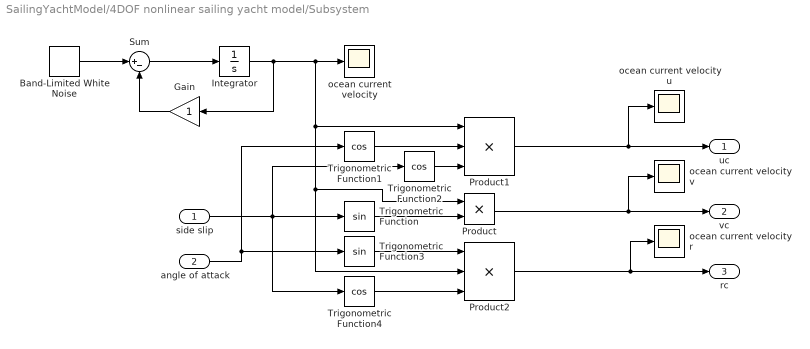
== system SailingYachtModel/4DOF nonlinear sailing yacht model/Subsystem ==
  side slip : Inport
  angle of attack : Inport  Port=2
  Band-Limited White Noise : simulink/Sources/Band-Limited White Noise  Cov=[0.05]  Ts=1  seed=[23341]
  Gain : Gain
  Integrator : Integrator
  Product : Product
  Product1 : Product  Inputs=3
  Product2 : Product  Inputs=3
  Sum : Sum  Inputs=|+-
  Trigonometric Function : Trigonometry
  Trigonometric Function1 : Trigonometry  Operator=cos
  Trigonometric Function2 : Trigonometry  Operator=cos
  Trigonometric Function3 : Trigonometry
  Trigonometric Function4 : Trigonometry  Operator=cos
  ocean current velocity : Scope
  ocean current velocity r : Scope
  ocean current velocity u : Scope
  ocean current velocity v : Scope
  uc : Outport
  vc : Outport  Port=2
  rc : Outport  Port=3
  wires:
  Sum/1 -> Integrator/1
  Band-Limited White Noise/1 -> Sum/1
  Integrator/1 -> Product1/1, Product2/2, Product/1, ocean current velocity/1, Gain/1
  Gain/1 -> Sum/2
  Trigonometric Function/1 -> Product/2
  side slip/1 -> Trigonometric Function4/1, Trigonometric Function2/1, Trigonometric Function/1
  Product/1 -> ocean current velocity v/1, vc/1
  Trigonometric Function2/1 -> Product1/3
  Trigonometric Function1/1 -> Product1/2
  Product1/1 -> ocean current velocity u/1, uc/1
  Trigonometric Function3/1 -> Product2/1
  Trigonometric Function4/1 -> Product2/3
  angle of attack/1 -> Trigonometric Function3/1, Trigonometric Function1/1
  Product2/1 -> rc/1, ocean current velocity r/1

== matlab function SailingYachtModel/MATLAB Function7 ==
  data: dist input; y output; xtrack input; angle output; currentState input; nextState output; ang input
function [y,angle,nextState]  = tackAngle(dist,xtrack,currentState,ang)
% Calculate when to tack back to waypoint
angle = atan(xtrack*cos(ang)/dist);
angle = angle * (180/pi);
nextState=1;
switch currentState
    case 0
        if angle>=52.5
        nextState=2;
        elseif angle<=-52.5
        nextState=1;
        else
        nextState=1;
        end
        y=0;

    case 1
        y = 1;
        if angle>=52.5
        nextState=2;
        else
            nextState=1;
        end

    case 2
        y=2;
        if angle<=-52.5
        nextState=1;
        else 
            nextState=2;
        end

    otherwise
        currentState=0;
        y=0;
end

== matlab function SailingYachtModel/MATLAB Function8 ==
  data: xs input; ys input; x input; y input; dist input; dist output
function dist   = travelDistance(xs,ys,x,y,dist)
% Distance Sailboat travelled

dist = dist + sqrt((xs-x)^2+(ys-y)^2);

== matlab function SailingYachtModel/4DOF nonlinear sailing yacht model/MATLAB Function ==
  data: u input; y output; s input; velocity input; su input; side input
function y = sailController(u,s,velocity,su,side)
% If s=1 traditional controller
% Else s=0 extreme seek sail controler
delta_sbar=pi/3;
if s==1
    y = u;
elseif s==0
    if velocity>0
        if side>0
        y=su+0.01;
        else
        y=su-0.01;
        end
        
        %Limit Sail Range
        if y > delta_sbar
            y = delta_sbar;
        elseif y <-delta_sbar
                y = -delta_sbar;
        end
    elseif velocity<0
        if side>0
        y=su-0.01;
        else
        y=su+0.01;
        end
        %Limit Sail Range
        if y > delta_sbar
            y = delta_sbar;
        elseif y <-delta_sbar
                y = -delta_sbar;
        end
    else
        y=su;
        %Limit Sail Range
        if y > delta_sbar
            y = delta_sbar;
        elseif y <-delta_sbar
                y = -delta_sbar;
        end
    end
else
    y=u;
end

== matlab function SailingYachtModel/MATLAB Function9 ==
  data: u input; y output; v input
function y  = correctAngle(u,v)
% Get the smallest angle between desired and actual heading
% Vector U (desired)
ux = cos(u);
uy = sin(u);

% Vector V (actual)
vx = cos(v);
vy = sin(v);

% Dot product u.v
dot = ux*vx + uy*vy;

% Vector Size
U = sqrt((ux)^2+(uy)^2);

V = sqrt((vx)^2+(vy)^2);
Size = U*V;

theta = acos(dot/Size);

y=theta;
u=u*180/pi;
v=v*180/pi;

if u<0
    u=u+180;
end

if v<0 
    v=v+360;
end

if (u-v)>180
    %y=-theta;
end

== matlab function SailingYachtModel/MATLAB Function10 ==
  data: state input; y output
function y = stopSimulation(state)
if state== 4
    y=1;
else
    y=0;
end

== matlab function SailingYachtModel/4DOF nonlinear sailing yacht model/MATLAB Function1 ==
  data: beta input; wu output; wv output; wr output; t input
function [wu,wv,wr] = WaveForcesandMoments(beta,t)
% Water density (kg/m^2)
rho = 1025;

% Gravity (m/s^2)
g = 9.81;

% Vessel size (m)
L = 12;
B = 3.12;
T = 1.85;

% Vessels Heading

% Wave Specifications
% amplitude(m)
Ai = 0.3;
% length(m)
lamdai = 10;
% encounter frequency (rads)
omegai = 0.4;
% random phase (rads)
phii = -pi;

% Wave Component
waveC = Ai * (2*pi)/lamdai * sin(omegai*t + phii);

% u Component
wu = (10^(-6)) * rho * g * B * L * T * cos(beta) * waveC;

% v Component
wv = (10^(-6)) * rho * g * B * L * T * sin(beta) * waveC;

% r Component
wr = (10^(-6)) * 1/24 * rho * g * B * L * (L^2 - B^2) * sin(2*beta) * waveC^2;

== matlab function SailingYachtModel/4DOF nonlinear sailing yacht model/MATLAB Function2 ==
  data: windDirect input; wi_u output; wi_v output; wi_r output; V_w input; psi input; u input; v input
function [wi_u,wi_v,wi_r] = WindForcesandMoments(windDirect,V_w,psi,u,v)
% Air density (kg/m^2)
rho = 1.225;

% Ship Size
L = 12;
B = 3.12;
T = 1.85;

% centroids above the water line of the frontal and lateral projected areas
H_fw = T - 1.2;
H_lw = T - 1.2;
A_fw = B * H_fw;
A_lw = L * H_lw;


% Symmetrical Ship Coeff
c_x = 0.7;
c_y = 0.825;
c_r = 0.125;

% Wind Velocities in x- and y-coordinates
u_w = V_w * cos(windDirect - psi);
v_w = V_w * sin(windDirect - psi);

% Relative wind velocities
u_rw = u - u_w;
v_rw = v - v_w;

% Relative Wind Velocity and direction
V_rw = sqrt(u_rw^2 + v_rw^2);
gamma_rw = -atan(v_rw/u_rw);

% Wind Coeff
C_x = -c_x * cos(gamma_rw);
C_y = c_y * sin(gamma_rw);
C_r = c_r * sin(2*gamma_rw);

% Wind Forces and Moments
wi_u = 0.5 * rho * V_rw *  C_x * A_fw * 10^(-2);
wi_v = 0.5 * rho * V_rw *  C_y * A_lw * 10^(-2);
wi_r = 0.5 * rho * V_rw *  C_r * A_lw * 10^(-2);

== matlab function SailingYachtModel/MATLAB Function11 ==
  data: xw input; yw input; xs input; p_w output; ys input; xcw input; ycw input; theta output
function [p_w,theta] = passedWaypoint(xw,yw,xs,ys,xcw,ycw)
% Checking is sailboat has passed waypoint while sailing into the wind
theta = atan(abs(xs-xcw)/abs(ys-ycw));
p_w=0;
if xw>0 
% Angle between sail
    if (xcw-xs)<0 
        % Waypoint passed in x positive
        p_w=1;
        if(ycw-ys)<0
            % Waypoint passed in both x and y positive direction
            theta = pi + theta;
        else
            % Waypoint passed in positive x and negative y
            theta = -theta;
        end
    end 
else
    if(xcw-xs)>0 
        % Waypoint passed in x negative
        p_w=1;
        if(ycw-ys)>0
           % Waypoint passed in both x and y negative direction
        else
           % Waypoint passed in negative x and positive y
           theta= pi - theta;
        end
   end
end

== matlab function SailingYachtModel/MATLAB Function1 ==
  data: tackHeading input; pathTrajectory input; y output; WA input; tack output; w_p input; tackDistance output; tackLeft output; tackRight output; wayPointHeading input; tackToWaypoint input; AWA output; theta_pw input; ys input
function [y,tack,tackDistance,tackLeft,tackRight,AWA]  = headingController(tackHeading,pathTrajectory,WA,w_p,wayPointHeading,tackToWaypoint,theta_pw,ys)
% Change wind angle to follow same convection as waypoint heading, ranges
% from -180 -> 180
theta_pw = theta_pw *180/pi;
if WA<0
   WA = WA + 360;
end
if wayPointHeading<0 
    wayPointHeading = wayPointHeading +360;
end
% Tack Direct==0 or Indirect==1
indirect=0;
% Apparent Wind Angle
AWA = wayPointHeading - WA;

% Determine the state of sailboat
if      abs(wayPointHeading-WA)<45
    % State 1: Tacking   
           % Initialize tacking right
           if(abs(tackHeading)<15)
                % Set tack angle to the right
                y=WA+60;
                % State value
                tack=0.5;
                % Tack Distance D
                tackDistance=15;
                % Tack Right Angle
                tackRight=WA+60;
                % Tack LEft Angle
                tackLeft=WA-60;
           elseif indirect==1
               % Reference heading
               y=WA-45;
               % State value
               tack=2;
               % Indirect Tack
               if tackToWaypoint == 1
                    y = WA+60;
               elseif tackToWaypoint == 2
                    y = WA-60;
               end
               tackDistance=15;
                % Tack Right Angle
                tackRight=WA+60;
                % Tack LEft Angle
                tackLeft=WA-60;
           else
               % Reference heading
               y=tackHeading;
               % State value
               tack=1;
               % Tack Right Angle
               tackRight=WA+60;
               % Tack LEft Angle
               tackLeft=WA-60;
               % Tack Distance D
               tackDistance=15;
           end
% State 0: Normal Sail 
else 
        % State Value
        tack=0;
        % Reference Heading
        y=pathTrajectory;
        % Reset tacking distance
        tackDistance=15;
        % Reset Right tack angle
        tackRight=WA+45;
        % Reset Left tack angle
        tackLeft=WA-45;
end
if w_p ==1 
    y = theta_pw;
    if (ys-w_p)>180
    y = theta_pw+360;
    end
end

== matlab function SailingYachtModel/MATLAB Function5 ==
  data: u input; y output
function y  = windAngle(u)
% Convert Wind Angle
x=u;
%if x>pi
    %y=x-2*pi;
%elseif x<-pi
    %y=x+2*pi;
%else
    %y=x;
%end
y=u;

== matlab function SailingYachtModel/MATLAB Function2 ==
  data: R input; nextState output; currentWaypoint output; currentState input
function [nextState,currentWaypoint]  = wayPointController(R,currentState)
% Waypoint switching
% With each added waypoint another case should be added
switch currentState
    % First waypoint
    case 0
        % Check if waypoint lies within radius of acceptance
        if(R==1)
            % Switch current Waypoint to next waypoint
            nextState=1;
            currentWaypoint=1;
        % Waypoint not reached
        else
            nextState=0;
            currentWaypoint=0;
        end
    case 1
        % Check if waypoint lies within radius of acceptance
        if(R==1)
            % Switch current Waypoint to next waypoint
            nextState=2;
            currentWaypoint=2;
       % Waypoint not reached
       else
            nextState=currentState;
            currentWaypoint=1;
       end
    case 2
       % Check if waypoint lies within radius of acceptance
       if(R==1)
            % Switch current Waypoint to next waypoint
            nextState=3;
            currentWaypoint=3;
       % Waypoint not reached
       else
            nextState=currentState;
            currentWaypoint=2;
       end
     case 3
       % Check if waypoint lies within radius of acceptance
       if(R==1)
            % Switch current Waypoint to next waypoint
            nextState=4;
            currentWaypoint=4;
       % Waypoint not reached 
       else
            nextState=currentState;
            currentWaypoint=3;
       end
     case 4
       % Check if waypoint lies within radius of acceptance
       if(R==1)
            % Switch current Waypoint to next waypoint
            nextState=0;
            currentWaypoint=0;
       % Waypoint not reached
       else
            nextState=currentState;
            currentWaypoint=4;
       end
    otherwise
        nextState=0;
        currentWaypoint=0;
end

== matlab function SailingYachtModel/MATLAB Function3 ==
  data: xWaypoint input; yWaypoint input; xBoat input; yBoat input; R input; acceptance output
function acceptance   = circleOfAcceptanceController(xWaypoint,yWaypoint,xBoat,yBoat,R)
    if (sqrt((abs(xWaypoint-xBoat))^2+(abs(yWaypoint-yBoat))^2)<R)
        acceptance=1;
    else
        acceptance=0;
    end
end

== matlab function SailingYachtModel/PID heading controller/MATLAB Function5 ==
  data: u input; y output; tack input
function y  = rudderGainP(u,tack)
% Check if sailboat is tacking
if tack==1
    y=-4*u;
else
    y=-1.5*u;
end

== matlab function SailingYachtModel/MATLAB Function4 ==
  data: xw input; yw input; xwp input; y output; ywp input
function y  = distanceToWaypoint(xw,yw,xwp,ywp)
% Calculate distance to waypoint
y = (sqrt((ywp-yw)^2+(xwp-xw)^2))/2;

== matlab function SailingYachtModel/MATLAB Function6 ==
  data: x1 input; y1 input; u input; y output; us input
function y = controlAngle(x1,y1,u,us)
ys=0;
if x1>=0 && y1>=0
    ys=u;
elseif x1>=0 && y1<=0
        ys=pi-u;
elseif x1==0 && y1>0
        ys=0;
elseif x1==0 && y1<0
        ys=pi;
elseif y1==0 && x1>0
        ys=pi/2;
elseif y1==0 && x1<0
        ys=-pi/2;
elseif x1<0 && y1>0
    ys=-u;
elseif x1<0 && y1<0
    ys=-pi+u;
else
    ys=u;
end
if (ys-us)<-pi
    y = ys+2*pi;
elseif (ys-us)>pi
    y=ys+2*pi;
else
    y=ys;
end
